simulink model "rosmca"  (Simulink 9.0)
settings: Solver=ode45  StartTime=0.0  StopTime=100  RelTol=1e-6  EnableMultiTasking=on
libraries: simulink x3
settings Model: Creator=Alli  LastModifiedBy=Matteo  ExtModeTrigMode=oneshot  ExtModeArmWhenConnect=off
settings DataIOCC: SignalLoggingSaveFormat=ModelDataLogs
settings OptimizationCC: BlockReduction=off  BooleanDataType=off  ExpressionDepthLimit=2147483647  InitFltsAndDblsToZero=on
settings DebuggingCC: SaveWithParameterizedLinksMsg=none  SignalResolutionControl=TryResolveAllWithWarning  MultiTaskDSMMsg=warning  MultiTaskCondExecSysMsg=none  FcnCallInpInsideContextMsg=warning  StateNameClashWarn=warning
settings HardwareCC: TargetUnknown=on
settings GRTTargetCC: GeneratePreprocessorConditionals=Disable all  CombineOutputUpdateFcns=off  GRTInterface=on

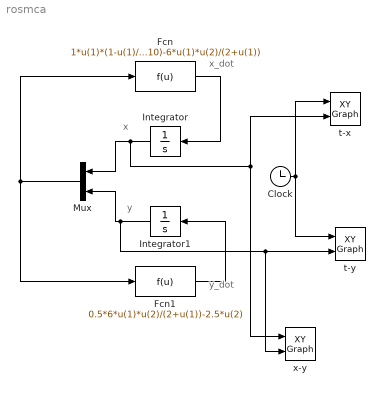
== system rosmca ==
  note: x_dot
  note: y_dot
  note: y
  note: x
  Clock : Clock
  Fcn : Fcn  Expr=1*u(1)*(1-u(1)/10)-6*u(1)*u(2)/(2+u(1))
  Fcn1 : Fcn  Expr=0.5*6*u(1)*u(2)/(2+u(1))-2.5*u(2)
  Integrator : Integrator  InitialCondition=4
  Integrator1 : Integrator  InitialCondition=2
  Mux : Mux  Inputs=2
  t-x : simulink/Sinks/XY Graph  xmin=0  xmax=100  ymin=0  ymax=12  st=0.01
  t-y : simulink/Sinks/XY Graph  xmin=0  xmax=100  ymin=0  ymax=4  st=0.01
  x-y : simulink/Sinks/XY Graph  xmin=0  xmax=12  ymin=0  ymax=4  st=0.01
  wires:
  Fcn/1 -> Integrator/1
  Fcn1/1 -> Integrator1/1
  Mux/1 -> Fcn/1, Fcn1/1
  Integrator/1 -> Mux/1, t-x/2, x-y/1
  Clock/1 -> t-x/1, t-y/1
  Integrator1/1 -> Mux/2, t-y/2, x-y/2
